simulink model "CPG_online"  (R2021b)
settings: Solver=FixedStepDiscrete  StartTime=0.0  StopTime=inf  FixedStep=Ts_cal  MaxStep=0.05  RelTol=0.5  AbsTol=0.5
model workspace (MATLAB code in the model file):
  | %---------------Critical values---------------%
  | angle_amp = pi/4; % Motor rotate amplitude, ref: pi/4
  | rotateCorrectionCoef = 1.158;
  | criticalFn = 2;
  | 
  | %------values for normalization---------------%
  | % values got by running manual gait
  | rotxNormGain = 1/0.1;
  | rotyNormGain = 1/0.05;
  | rotzNormGain = 1/0.1;
  | 
  | vxNormGain = 1/0.2;
  | vyNormGain = 1/0.2;
  | vzNormGain = 1/0.2;
  | 
  | FnNormGain = 1/15;
  | 
  | %--------values for check done---------------%
  | rotDone = pi/6;
  | legBendDone = pi/3; % actuator max bending angle
  | 
  | %---------------Robot parameters-------------%
  | % robot size
  | robot_width = 0.15;
  | robot_length = 0.22;
  | 
  | % floor parameters
  | floor_length = 2;
  | floor_width = 2;
  | 
  | % continuum actuator size
  | L_disk = 0.02944;% Disk side length (m)
  | R_w = L_disk/sqrt(3);
  | thickness_disk = 0.004; % Disk thickness (m)
  | thigh_length = 0.06;
  | R_core = 0.005; % Core radius (m)
  | length_core = 0.008; % Core length (m)
  | R_spool = 0.021; % 0.01944; % radius of the spool
  | spool_height = 0.022+0.015;
  | R_pulley = 1e-3;
  | spool_k = 0;
  | spool_d = 0;
  | hole_d = 4e-3;
  | 
  | % Material property
  | rho_PLA = 1.24e3;
  | rho = 1.19e3; % 1.19e3; % Density (kg/m^3)
  | % use rigid joints
  | Pz_stiff = 135000;
  | Pz_damping = 500;
  | S_stiff = 0.0239;
  | S_damping = 7.5e-5;
  | S_low_Bound = -20;
  | S_up_Bound = 20;
  | 
  | R_foot = 0.015; % foot radius (m)
  | 
  | % motor parameter
  | stall_T = 11.2/10; % 11.2 cm*kg, stall torque
  | t_60_deg = 0.2; % 0.09 s
  | V_nomrmal = 6; % corresponding normal voltage
  | Jr = 0.0001; %g*cm^2, robot inertia
  | 
  | % contact force
  | coef_static_friction = 0.315;
  | coef_dynamic_friction = 0.3;
  | crictic_velocity = 0.3; % m/s
  | contact_suf_stiff = 1000; % N/m
  | contact_suf_damp = 50; % N/(m/s)
  | contact_region_width = 2e-3; % m
  | spoolOpacity = 0;
  | tendonColor = [0.902 0.902 0.902];
  | tendonOpacity = 0.1;
  | 
  | % If use point masses
  | MMainFrame = 198; % g
  | MServoMotor = 50.55;
  | MMotorSupport = 12.1;
  | MSpool = 9.2;
  | 
  | % Robot total weight about 2 kg
  | MComposateLoad = 200;
  | 
  | MBuck = 40; % x2
  | MPCB_RPi = 141.3;
  | MLiBattery = 120; % x2
  | MPowerBank = 66.5;
  | isLoadVisible = 0.1;
  | 
  | 
  | MThigh = 26.7963;
  | MCore = 0.747699;
  | MDisk = 1.78642;
  | MFoot = 16.8232;
values from neighbouring files (symbols this model uses):
  A = [0 Ts; 0 1]    [MFBO_main.m]    (also in MFGP_main.m)
  A_cpg = 1    [MFBO_main.m]    (also in MFGP_main.m)
  alpha = opt_param(2)    [MFBO_main.m]    (also in MFGP_main.m)
  alpha_b_gain = opt_param(3)    [MFBO_main.m]    (also in MFGP_main.m)
  alpha_r_gain = pi    (= 3.14159265359)    [MFBO_main.m]    (also in MFGP_main.m)
  B = [0.5*Ts^2; Ts]    [MFBO_main.m]    (also in MFGP_main.m)
  C = [1 0]    [MFBO_main.m]    (also in MFGP_main.m)
  epsilon = 5    [MFBO_main.m]    (also in MFGP_main.m)
  f = 1/T    [MFBO_main.m]    (also in MFGP_main.m)
  init_state = rand(1, 8)*2 - 1    [MFBO_main.m]    (also in MFGP_main.m)
  k = 1000    [MFBO_main.m]    (also in MFGP_main.m)
  phi_vec = pi*[-1; 1; -1; 1]    [MFBO_main.m]    (also in MFGP_main.m)
  R = 0.15    [MFBO_main.m]    (also in MFGP_main.m)
  tau = 1    [MFBO_main.m]    (also in MFGP_main.m)
  Ts = 5e-2    (= 0.05)    [MFBO_main.m]    (also in MFGP_main.m)
  Ts_cal = 5e-4    (= 0.0005)    [MFBO_main.m]    (also in MFGP_main.m)
  z_l_diff = opt_param(5)    [MFBO_main.m]    (also in MFGP_main.m)
  z_l_gain = opt_param(4)    [MFBO_main.m]    (also in MFGP_main.m)
undefined symbols (not defined in the file or in its folder): DiscIntNeverNeededParam, Discrete, Time
libraries: svdutilitieslib x15, simulink x4, ctrlSharedLib x3, instrumentlib x2, aerolibanimutils x1
(part 1 of 2)
settings Model: Creator=Qinglei Ji  LastModifiedBy=4DLab5
settings SolverCC: AutoScaleAbsTol=off  MaxConsecutiveZCs=100  MaxConsecutiveMinStep=10  DaesscMode=Fast  ZeroCrossAlgorithm=Adaptive  AutoInsertRateTranBlk=on
settings DebuggingCC: AlgebraicLoopMsg=error  IgnoredZcDiagnostic=none
settings ExplorerConfigSet: InternalSimMechanicsExplorerSettings="<ExplorerConfiguration><canonicalview>default</canonicalview><AnimationSetting><BasePlaybackSpeed>1.0</BasePlaybackSpeed><PlaybackSpeedFactor>1.0</PlaybackSpeedFactor></AnimationSetting><TilePanel><TileInfo><Tiles Columns=\"1\" Count=\"1\" Rows=\"1\"><Column Weight=\"1\"/><Row Weight=\"1\"/><Tile Height=\"1\" Width=\"1\" X=\"0\" Y=\"0\"/></Tiles></TileInfo><SceneInfo><SceneViewer><BGColor><R>0.60000002384185791</R><G>0.60000002384185791</G><B>0.60000002384185791</B></BGColor><Camera><DoPerspective>off</DoPerspective><Position><X>-18.8331461547739707</X><Y>25.880517186070815</Y><Z>26.8100820833696147</Z></Position><Center><X>0.29785977478998571</X><Y>-0.293010908258582892</Y><Z>-0.346783787749327221</Z></Center><Up><X>0.517886432622382209</X><Y>-0.40389178028612327</Y><Z>0.754098848111419029</Z></Up><ViewLimDist>1</ViewLimDist><YLim>0.421333194645766129</YLim><XLim>0.456755011894746488</XLim></Camera></SceneViewer></SceneInfo></TilePanel><MechEditorPanel><Cameras/><GfxPanelCameraMap/><VideoCreator><PlaybackSpeedRatio>1.0</PlaybackSpeedRatio><FrameRate>60</FrameRate><VideoFormat>MPEG-4</VideoFormat><FrameSize>auto</FrameSize></VideoCreator></MechEditorPanel></ExplorerConfiguration>"

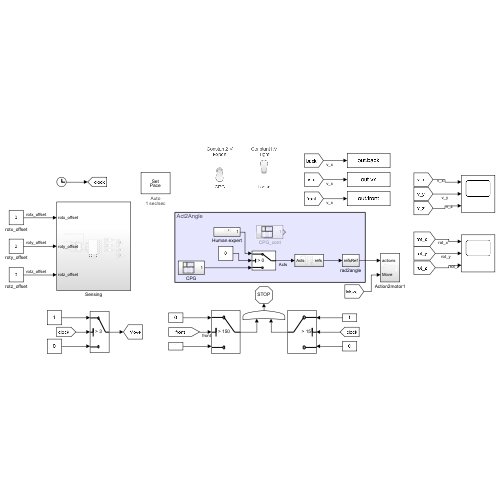
[thumbnail: Simulink's stored preview of the top-level diagram]
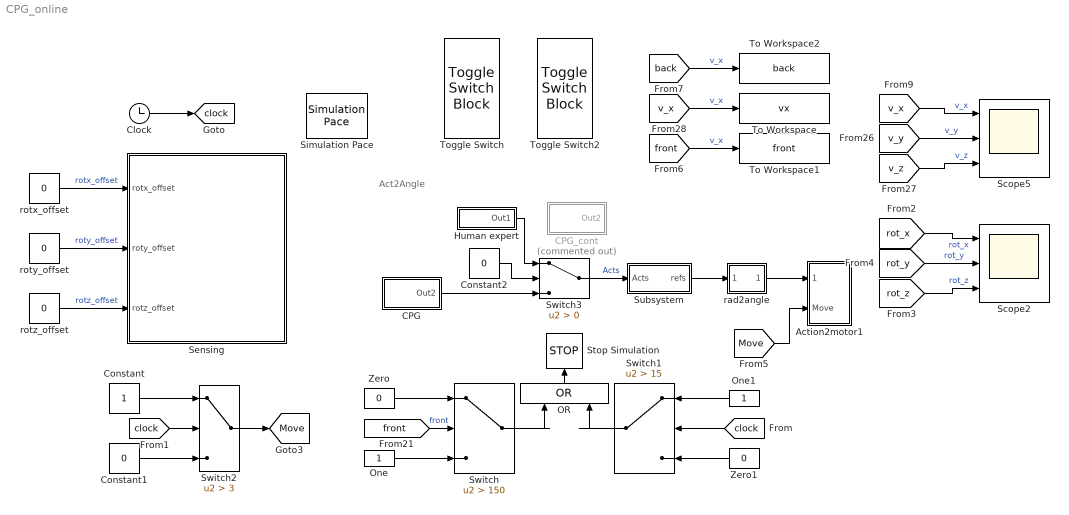
== system CPG_online ==
  note: Act2Angle
  Action2motor1 : Subsystem
  CPG : Subsystem
  CPG_cont : Subsystem  Commented=on
  Clock : Clock
  Constant : Constant
  Constant1 : Constant  Value=0
  Constant2 : Constant  Value=0
  Human expert : Subsystem
  OR : Logic  Operator=OR  IconShape=distinctive  AllPortsSameDT=off  OutDataTypeStr=boolean
  One : Constant  OutDataTypeStr=Inherit: Inherit via back propagation
  One1 : Constant  OutDataTypeStr=Inherit: Inherit via back propagation
  Scope2 : Scope  NumInputPorts=3
  Scope5 : Scope  NumInputPorts=3
  Sensing : Subsystem
  Simulation Pace : aerolibanimutils/Simulation Pace  SimulationPace=1  SleepMode=Auto  OutputPaceError=off  SampleTime=0.05
  Stop Simulation : Stop
  Subsystem : Subsystem
  Switch : Switch  Criteria=u2 > Threshold  Threshold=150
  Switch1 : Switch  Criteria=u2 > Threshold  Threshold=15
  Switch2 : Switch  Criteria=u2 > Threshold  Threshold=3
  Switch3 : Switch  Criteria=u2 > Threshold
  To Workspace : ToWorkspace  VariableName=vx  SampleTime=-1
  To Workspace1 : ToWorkspace  VariableName=front  SampleTime=-1
  To Workspace2 : ToWorkspace  VariableName=back  SampleTime=-1
  Toggle Switch : ToggleSwitchBlock
      settings: Values={{'CPG', 'Expert'}, [0 1]}
  Toggle Switch2 : ToggleSwitchBlock
      settings: Values={{'Loose', 'Tight'}, [0 1]}
  Zero : Constant  Value=0  OutDataTypeStr=Inherit: Inherit via back propagation
  Zero1 : Constant  Value=0  OutDataTypeStr=Inherit: Inherit via back propagation
  rad2angle : Subsystem
  rotx_offset : Constant  Value=0
  roty_offset : Constant  Value=0
  rotz_offset : Constant  Value=0
  tag scope: Move=global, clock=global
  wires:
  rad2angle/1(Ref) -> Action2motor1/1(actions)
  OR/1 -> Stop Simulation/1
  [front] -> Switch/2  "front"
  Zero/1 -> Switch/1
  One/1 -> Switch/3
  Switch/1 -> OR/1
  Switch1/1 -> OR/2
  Clock/1 -> [clock]
  [clock] -> Switch1/2
  Zero1/1 -> Switch1/3
  One1/1 -> Switch1/1
  [rot_y] -> Scope2/2  "rot_y"
  [rot_z] -> Scope2/3  "rot_z"
  [rot_x] -> Scope2/1  "rot_x"
  [v_z] -> Scope5/3  "v_z"
  [v_y] -> Scope5/2  "v_y"
  [v_x] -> Scope5/1  "v_x"
  [v_x] -> To Workspace/1  "v_x"
  Subsystem/1(refs) -> rad2angle/1(refs)
  Switch3/1 -> Subsystem/1(Acts)  "Acts"
  rotx_offset/1 -> Sensing/1(rotx_offset)  "rotx_offset"
  roty_offset/1 -> Sensing/2(roty_offset)  "roty_offset"
  rotz_offset/1 -> Sensing/3(rotz_offset)  "rotz_offset"
  Constant/1 -> Switch2/1
  Constant1/1 -> Switch2/3
  [clock] -> Switch2/2
  Switch2/1 -> [Move]
  [Move] -> Action2motor1/2(Move)
  Constant2/1 -> Switch3/2
  Human expert/1(Out1) -> Switch3/1
  CPG/1(Out2) -> Switch3/3
  [front] -> To Workspace1/1  "v_x"
  [back] -> To Workspace2/1  "v_x"

== system CPG_online/Action2motor1 ==
  actions : Inport
  Move : Inport  Port=2
  Add : Sum  Inputs=+-
  Constant : Constant  Value=0
  Constant1 : Constant
  Constant2 : Constant  Value=15
  Data Type Conversion2 : DataTypeConversion  OutDataTypeStr=uint8
  Display : Display
  Rate Transition : RateTransition  OutPortSampleTime=Ts
  Switch : Switch  Criteria=u2 > Threshold
  Switch1 : Switch  Criteria=u2 > Threshold
  TCP/IP Send : instrumentlib/TCP//IP Send  Priority=1  Host=192.168.0.111  Port=6666  ByteOrder=big-endian  EnableBlockingMode=on  Timeout=1  TransferDelay=on  SimulateUsing=Interpreted execution
  manual angle input2 : Subsystem
  pretighten : Subsystem
  pretighten1 : Subsystem  Commented=on
  wires:
  manual angle input2/1(Out1) -> Switch1/3
  pretighten/1(Out1) -> Add/2
  Switch1/1 -> Add/1
  Switch/1 -> pretighten/1(In1)
  Constant/1 -> Switch/3
  Constant2/1 -> Switch/1
  Data Type Conversion2/1 -> Display/1, TCP/IP Send/1
  Add/1 -> Rate Transition/1
  Constant1/1 -> Switch/2
  Move/1 -> Switch1/2
  actions/1 -> Switch1/1
  Rate Transition/1 -> Data Type Conversion2/1

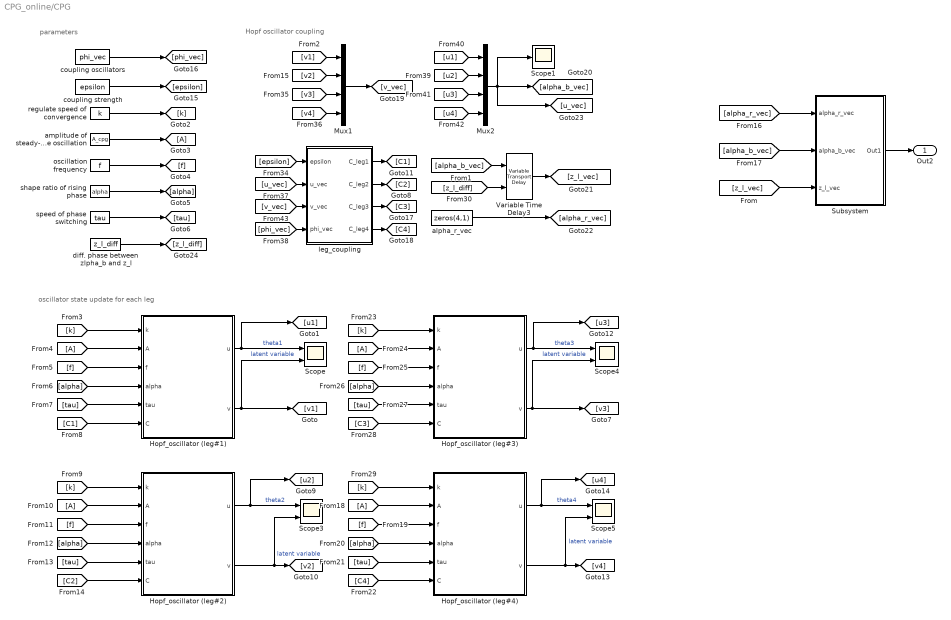
== system CPG_online/CPG ==
  note: oscillator state update for each leg
  note: Hopf oscillator coupling
  note: parameters
  Hopf_oscillator (leg#1) : Subsystem
  Hopf_oscillator (leg#2) : Subsystem
  Hopf_oscillator (leg#3) : Subsystem
  Hopf_oscillator (leg#4) : Subsystem
  Mux1 : Mux
  Mux2 : Mux
  Scope{,3..5} (4 alike) : Scope  NumInputPorts=2
  Scope1 : Scope
  Subsystem : Subsystem
  Variable Time Delay3 : VariableTransportDelay  MaximumDelay=10  MaximumPoints=2^20  FixedBuffer=on  ZeroDelay=on
  alpha_r_vec : Constant  Value=zeros(4,1)
  amplitude of steady-state oscillation : Constant  Value=A_cpg
  coupling oscillators : Constant  Value=phi_vec
  coupling strength : Constant  Value=epsilon
  diff. phase between zlpha_b and z_l : Constant  Value=z_l_diff
  leg_coupling : MATLAB Function  TreatAsAtomicUnit=on
  oscillation frequency : Constant  Value=f
  regulate speed of convergence : Constant  Value=k
  shape ratio of rising phase : Constant  Value=alpha
  speed of phase switching : Constant  Value=tau
  Out2 : Outport
  wires:
  [k] -> Hopf_oscillator (leg#4)/1(k)
  [tau] -> Hopf_oscillator (leg#3)/5(tau)
  [u4] -> Mux2/4
  [v2] -> Mux1/2
  shape ratio of rising phase/1 -> [alpha]
  [epsilon] -> leg_coupling/1(epsilon)
  [u3] -> Mux2/3
  [v_vec] -> leg_coupling/3(v_vec)
  [C2] -> Hopf_oscillator (leg#2)/6(C)
  leg_coupling/4(C_leg4) -> [C4]
  [f] -> Hopf_oscillator (leg#3)/3(f)
  Hopf_oscillator (leg#4)/1(u) -> [u4], Scope5/1  "theta4"
  Hopf_oscillator (leg#4)/2(v) -> [v4], Scope5/2  "latent variable"
  [k] -> Hopf_oscillator (leg#3)/1(k)
  leg_coupling/2(C_leg2) -> [C2]
  oscillation frequency/1 -> [f]
  [u1] -> Mux2/1
  Hopf_oscillator (leg#3)/1(u) -> [u3], Scope4/1  "theta3"
  [A] -> Hopf_oscillator (leg#3)/2(A)
  leg_coupling/3(C_leg3) -> [C3]
  [u2] -> Mux2/2
  Hopf_oscillator (leg#1)/2(v) -> [v1], Scope/2  "latent variable"
  [alpha] -> Hopf_oscillator (leg#2)/4(alpha)
  Hopf_oscillator (leg#3)/2(v) -> [v3], Scope4/2  "latent variable"
  speed of phase switching/1 -> [tau]
  [f] -> Hopf_oscillator (leg#2)/3(f)
  [tau] -> Hopf_oscillator (leg#4)/5(tau)
  [u_vec] -> leg_coupling/2(u_vec)
  [alpha] -> Hopf_oscillator (leg#3)/4(alpha)
  amplitude of steady-state oscillation/1 -> [A]
  [A] -> Hopf_oscillator (leg#1)/2(A)
  [A] -> Hopf_oscillator (leg#2)/2(A)
  leg_coupling/1(C_leg1) -> [C1]
  Mux2/1 -> [u_vec], [alpha_b_vec], Scope1/1
  Hopf_oscillator (leg#2)/1(u) -> [u2], Scope3/1  "theta2"
  [v4] -> Mux1/4
  [f] -> Hopf_oscillator (leg#4)/3(f)
  [C4] -> Hopf_oscillator (leg#4)/6(C)
  [C3] -> Hopf_oscillator (leg#3)/6(C)
  [tau] -> Hopf_oscillator (leg#1)/5(tau)
  coupling strength/1 -> [epsilon]
  [A] -> Hopf_oscillator (leg#4)/2(A)
  [k] -> Hopf_oscillator (leg#2)/1(k)
  [alpha] -> Hopf_oscillator (leg#4)/4(alpha)
  [v3] -> Mux1/3
  [k] -> Hopf_oscillator (leg#1)/1(k)
  [phi_vec] -> leg_coupling/4(phi_vec)
  [C1] -> Hopf_oscillator (leg#1)/6(C)
  [v1] -> Mux1/1
  Mux1/1 -> [v_vec]
  [tau] -> Hopf_oscillator (leg#2)/5(tau)
  [f] -> Hopf_oscillator (leg#1)/3(f)
  regulate speed of convergence/1 -> [k]
  Hopf_oscillator (leg#2)/2(v) -> [v2], Scope3/2  "latent variable"
  Hopf_oscillator (leg#1)/1(u) -> [u1], Scope/1  "theta1"
  [alpha] -> Hopf_oscillator (leg#1)/4(alpha)
  coupling oscillators/1 -> [phi_vec]
  [alpha_b_vec] -> Variable Time Delay3/1
  [z_l_diff] -> Variable Time Delay3/2
  Variable Time Delay3/1 -> [z_l_vec]
  alpha_r_vec/1 -> [alpha_r_vec]
  [alpha_r_vec] -> Subsystem/1(alpha_r_vec)
  [alpha_b_vec] -> Subsystem/2(alpha_b_vec)
  [z_l_vec] -> Subsystem/3(z_l_vec)
  Subsystem/1(Out1) -> Out2/1
  diff. phase between zlpha_b and z_l/1 -> [z_l_diff]

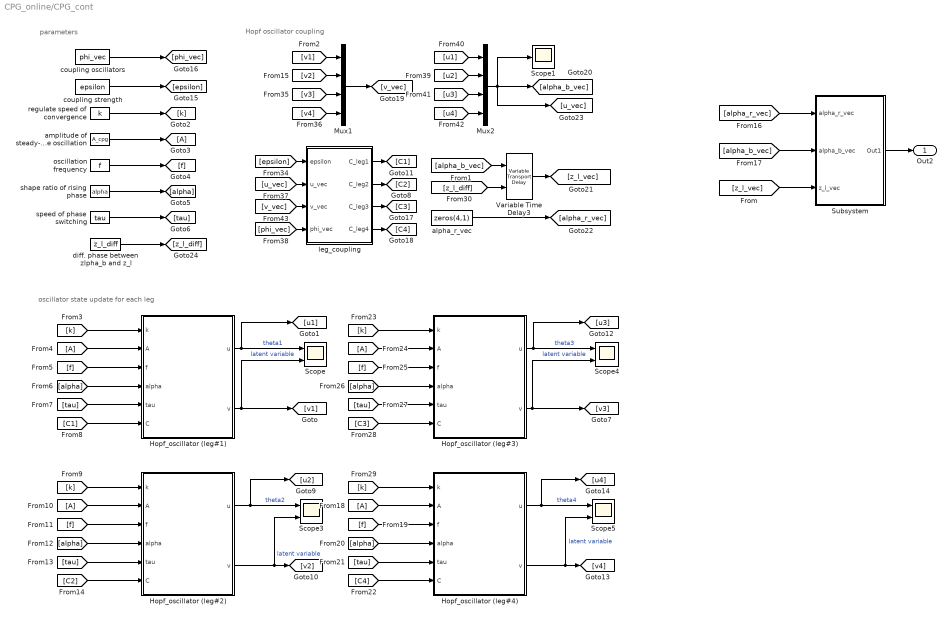
== system CPG_online/CPG_cont ==
  note: oscillator state update for each leg
  note: Hopf oscillator coupling
  note: parameters
  Hopf_oscillator (leg#1) : Subsystem
  Hopf_oscillator (leg#2) : Subsystem
  Hopf_oscillator (leg#3) : Subsystem
  Hopf_oscillator (leg#4) : Subsystem
  Mux1 : Mux
  Mux2 : Mux
  Scope{,3..5} (4 alike) : Scope  NumInputPorts=2
  Scope1 : Scope
  Subsystem : Subsystem
  Variable Time Delay3 : VariableTransportDelay  MaximumDelay=10  MaximumPoints=4096  ZeroDelay=on
  alpha_r_vec : Constant  Value=zeros(4,1)
  amplitude of steady-state oscillation : Constant  Value=A_cpg
  coupling oscillators : Constant  Value=phi_vec
  coupling strength : Constant  Value=epsilon
  diff. phase between zlpha_b and z_l : Constant  Value=z_l_diff
  leg_coupling : MATLAB Function  TreatAsAtomicUnit=on
  oscillation frequency : Constant  Value=f
  regulate speed of convergence : Constant  Value=k
  shape ratio of rising phase : Constant  Value=alpha
  speed of phase switching : Constant  Value=tau
  Out2 : Outport
  wires:
  [k] -> Hopf_oscillator (leg#4)/1(k)
  [tau] -> Hopf_oscillator (leg#3)/5(tau)
  [u4] -> Mux2/4
  [v2] -> Mux1/2
  shape ratio of rising phase/1 -> [alpha]
  [epsilon] -> leg_coupling/1(epsilon)
  [u3] -> Mux2/3
  [v_vec] -> leg_coupling/3(v_vec)
  [C2] -> Hopf_oscillator (leg#2)/6(C)
  leg_coupling/4(C_leg4) -> [C4]
  [f] -> Hopf_oscillator (leg#3)/3(f)
  Hopf_oscillator (leg#4)/1(u) -> [u4], Scope5/1  "theta4"
  Hopf_oscillator (leg#4)/2(v) -> [v4], Scope5/2  "latent variable"
  [k] -> Hopf_oscillator (leg#3)/1(k)
  leg_coupling/2(C_leg2) -> [C2]
  oscillation frequency/1 -> [f]
  [u1] -> Mux2/1
  Hopf_oscillator (leg#3)/1(u) -> [u3], Scope4/1  "theta3"
  [A] -> Hopf_oscillator (leg#3)/2(A)
  leg_coupling/3(C_leg3) -> [C3]
  [u2] -> Mux2/2
  Hopf_oscillator (leg#1)/2(v) -> [v1], Scope/2  "latent variable"
  [alpha] -> Hopf_oscillator (leg#2)/4(alpha)
  Hopf_oscillator (leg#3)/2(v) -> [v3], Scope4/2  "latent variable"
  speed of phase switching/1 -> [tau]
  [f] -> Hopf_oscillator (leg#2)/3(f)
  [tau] -> Hopf_oscillator (leg#4)/5(tau)
  [u_vec] -> leg_coupling/2(u_vec)
  [alpha] -> Hopf_oscillator (leg#3)/4(alpha)
  amplitude of steady-state oscillation/1 -> [A]
  [A] -> Hopf_oscillator (leg#1)/2(A)
  [A] -> Hopf_oscillator (leg#2)/2(A)
  leg_coupling/1(C_leg1) -> [C1]
  Mux2/1 -> [u_vec], [alpha_b_vec], Scope1/1
  Hopf_oscillator (leg#2)/1(u) -> [u2], Scope3/1  "theta2"
  [v4] -> Mux1/4
  [f] -> Hopf_oscillator (leg#4)/3(f)
  [C4] -> Hopf_oscillator (leg#4)/6(C)
  [C3] -> Hopf_oscillator (leg#3)/6(C)
  [tau] -> Hopf_oscillator (leg#1)/5(tau)
  coupling strength/1 -> [epsilon]
  [A] -> Hopf_oscillator (leg#4)/2(A)
  [k] -> Hopf_oscillator (leg#2)/1(k)
  [alpha] -> Hopf_oscillator (leg#4)/4(alpha)
  [v3] -> Mux1/3
  [k] -> Hopf_oscillator (leg#1)/1(k)
  [phi_vec] -> leg_coupling/4(phi_vec)
  [C1] -> Hopf_oscillator (leg#1)/6(C)
  [v1] -> Mux1/1
  Mux1/1 -> [v_vec]
  [tau] -> Hopf_oscillator (leg#2)/5(tau)
  [f] -> Hopf_oscillator (leg#1)/3(f)
  regulate speed of convergence/1 -> [k]
  Hopf_oscillator (leg#2)/2(v) -> [v2], Scope3/2  "latent variable"
  Hopf_oscillator (leg#1)/1(u) -> [u1], Scope/1  "theta1"
  [alpha] -> Hopf_oscillator (leg#1)/4(alpha)
  coupling oscillators/1 -> [phi_vec]
  [alpha_b_vec] -> Variable Time Delay3/1
  [z_l_diff] -> Variable Time Delay3/2
  Variable Time Delay3/1 -> [z_l_vec]
  alpha_r_vec/1 -> [alpha_r_vec]
  [alpha_r_vec] -> Subsystem/1(alpha_r_vec)
  [alpha_b_vec] -> Subsystem/2(alpha_b_vec)
  [z_l_vec] -> Subsystem/3(z_l_vec)
  Subsystem/1(Out1) -> Out2/1
  diff. phase between zlpha_b and z_l/1 -> [z_l_diff]

== system CPG_online/Human expert ==
  Constant : Constant  Value=0+0.4  SampleTime=Ts
  Constant1 : Constant  Value=0  SampleTime=Ts
  Constant2 : Constant  Value=0+0.4  SampleTime=Ts
  Mux1 : Mux  Inputs=3
  Mux2 : Mux
  Mux3 : Mux  Commented=on  Inputs=3
  Sine Wave : Sin  Frequency=2*pi/0.8  SampleTime=Ts
  Sine Wave1 : Sin  Frequency=2*pi/0.8  Phase=pi  SampleTime=Ts
  Variable Time Delay : VariableTransportDelay  MaximumDelay=10  MaximumPoints=2^15  ZeroDelay=on
  Variable Time Delay1 : VariableTransportDelay  MaximumDelay=10  MaximumPoints=2^15  ZeroDelay=on
  Variable Time Delay2 : VariableTransportDelay  MaximumDelay=10  MaximumPoints=2^15  ZeroDelay=on
  alpha_b : simulink/Sources/Repeating Sequence  Commented=on  rep_seq_t=[0 0.2 0.4 0.6 0.8]  rep_seq_y=[0 1 0 -1 0]
  alpha_b1 : simulink/Sources/Repeating Sequence  Commented=on  rep_seq_t=[0 0.2 0.4 0.6 0.8]  rep_seq_y=[0 -1 0 1 0]
  alpha_r : Constant  Value=0
  alpha_r1 : Constant  Commented=on  Value=0
  z_l : simulink/Sources/Repeating Sequence  Commented=on  rep_seq_t=[0 0.2 0.4 0.6 0.8]  rep_seq_y=[-1 1 1 1 -1]
  z_l1 : simulink/Sources/Repeating Sequence  Commented=on  rep_seq_t=[0 0.2 0.4 0.6 0.8]  rep_seq_y=[1 1 -1 1 1]
  Out1 : Outport
  wires:
  Mux2/1 -> Out1/1
  Mux1/1 -> Variable Time Delay2/1, Variable Time Delay/1, Mux2/1, Variable Time Delay1/1
  Sine Wave/1 -> Mux1/2  "alpha_b_Ref"
  alpha_r/1 -> Mux1/1  "alpha_r_Ref"
  Sine Wave1/1 -> Mux1/3  "z_l_Ref"
  Constant/1 -> Variable Time Delay/2
  z_l1/1 -> Mux3/3  "z_l_Ref"
  alpha_r1/1 -> Mux3/1  "alpha_r_Ref"
  alpha_b1/1 -> Mux3/2  "alpha_b_Ref"
  Variable Time Delay/1 -> Mux2/2
  Constant1/1 -> Variable Time Delay1/2
  Variable Time Delay2/1 -> Mux2/4
  Variable Time Delay1/1 -> Mux2/3
  Constant2/1 -> Variable Time Delay2/2

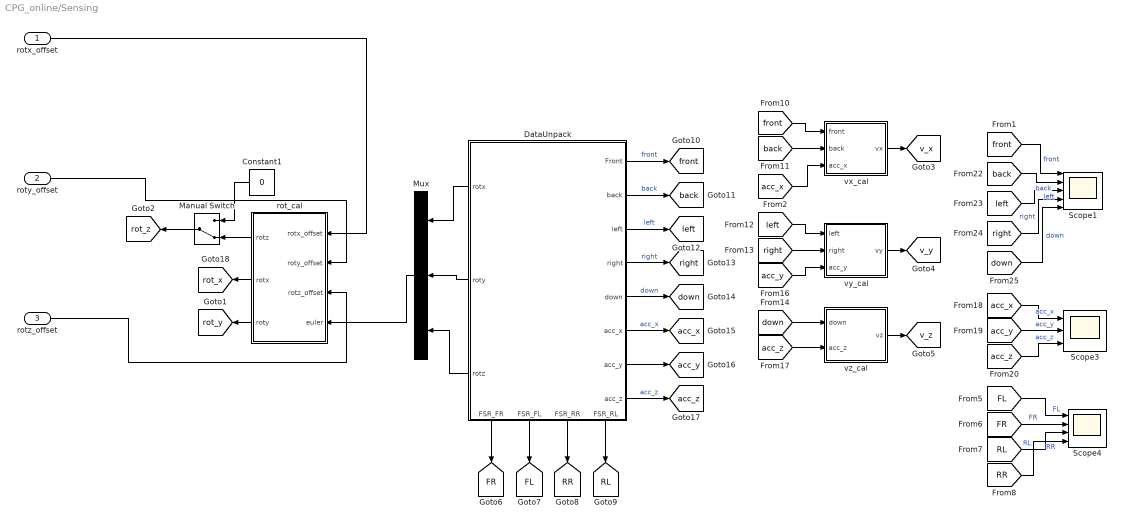
== system CPG_online/Sensing ==
  rotx_offset : Inport
  roty_offset : Inport  Port=2
  rotz_offset : Inport  Port=3
  Constant1 : Constant  Value=0
  DataUnpack : Subsystem
      settings: PortSchema="{\"entries\":[{\"content\":{\"sides\":[{\"content\":{\"connectorIds\":[\"Out13\",\"Out14\",\"Out15\"]},\"type\":\"ConnectorPlacement.EquallySpacedRectSide\",\"uuid\":\"921b036b-a103-4c29-98a4-1e13be366f27\"},{\"content\":{\"connectorIds\":[\"Out1\",\"Out2\",\"Out3\",\"Out4\",\"Out5\",\"Out6\",\"Out7\",\"Out8\"],\"side\":\"RIGHT\"},\"type\":\"ConnectorPlacement.EquallySpacedRectSide\",\"uuid\":\"743cc973-2ca6-4eb4-ab94-a827ba3cd866\"},{\"content\":{\"side\":\"TOP\"},\"type\":\"ConnectorPlacement.EquallySpacedRectSide\",\"uuid\":\"9eb642df-d260-4317-8a72-bd8569bebf98\"},{\"content\":{\"connectorIds\":[\"Out9\",\"Out10\",\"Out11\",\"Out12\"],\"side\":\"BOTTOM\"},\"type\":\"ConnectorPlacement.EquallySpacedRectSide\",\"uuid\":\"da7ab237-c829-42b0-bbc7-f99a364eb64c\"}]},\"type\":\"ConnectorPlacement.EquallySpacedConnector\",\"uuid\":\"aa8a793e-4baf-4a67-be1f-284a705b408b\"}],\"packageUris\":[\"http://schema.mathworks.com/mf0/Connector/R2020b\"],\"version\":\"1.0\"}"
  Manual Switch : ManualSwitch  CurrentSetting=0
  Mux : Mux  Inputs=3
  Scope1 : Scope  NumInputPorts=5
  Scope3 : Scope  NumInputPorts=3
  Scope4 : Scope  NumInputPorts=4
  rot_cal : Subsystem
  vx_cal : Subsystem
  vy_cal : Subsystem
  vz_cal : Subsystem
  tag scope: FL=global, FR=global, RL=global, RR=global, acc_x=global, acc_y=global, acc_z=global, back=global, down=global, front=global, left=global, right=global, rot_x=global, rot_y=global, rot_z=global, v_x=global, v_y=global, v_z=global
  wires:
  DataUnpack/10(FSR_FL) -> [FL]
  DataUnpack/4(right) -> [right]  "right"
  [RR] -> Scope4/4  "RR"
  [acc_y] -> Scope3/2  "acc_y"
  [FR] -> Scope4/2  "FR"
  [back] -> Scope1/2  "back"
  [RL] -> Scope4/3  "RL"
  [front] -> Scope1/1  "front"
  [front] -> vx_cal/1(front)
  DataUnpack/2(back) -> [back]  "back"
  DataUnpack/11(FSR_RR) -> [RR]
  [FL] -> Scope4/1  "FL"
  [right] -> Scope1/4  "right"
  rot_cal/3(roty) -> [rot_y]
  rot_cal/1(rotz) -> Manual Switch/2
  DataUnpack/12(FSR_RL) -> [RL]
  DataUnpack/8(acc_z) -> [acc_z]  "acc_z"
  rotx_offset/1 -> rot_cal/1(rotx_offset)
  vy_cal/1(vy) -> [v_y]
  DataUnpack/9(FSR_FR) -> [FR]
  DataUnpack/7(acc_y) -> [acc_y]
  Mux/1 -> rot_cal/4(euler)
  DataUnpack/15(rotz) -> Mux/3
  DataUnpack/6(acc_x) -> [acc_x]  "acc_x"
  DataUnpack/13(rotx) -> Mux/1
  DataUnpack/14(roty) -> Mux/2
  vz_cal/1(vz) -> [v_z]
  [back] -> vx_cal/2(back)
  DataUnpack/5(down) -> [down]  "down"
  DataUnpack/3(left) -> [left]  "left"
  DataUnpack/1(Front) -> [front]  "front"
  rotz_offset/1 -> rot_cal/3(rotz_offset)
  [acc_x] -> Scope3/1  "acc_x"
  [acc_z] -> Scope3/3  "acc_z"
  Manual Switch/1 -> [rot_z]
  Constant1/1 -> Manual Switch/1
  rot_cal/2(rotx) -> [rot_x]
  vx_cal/1(vx) -> [v_x]
  [left] -> Scope1/3  "left"
  [down] -> Scope1/5  "down"
  [acc_z] -> vz_cal/2(acc_z)
  [acc_y] -> vy_cal/3(acc_y)
  [right] -> vy_cal/2(right)
  roty_offset/1 -> rot_cal/2(roty_offset)
  [down] -> vz_cal/1(down)
  [left] -> vy_cal/1(left)
  [acc_x] -> vx_cal/3(acc_x)

== system CPG_online/Subsystem ==
  Acts : Inport
  Demux : Demux
  FL : Subsystem
  FR : Subsystem
  Mux : Mux
  RL : Subsystem
  RR : Subsystem
  To Workspace : ToWorkspace  VariableName=action  SaveFormat=Structure  SampleTime=Ts
      settings: Save2DSignal=2-D array (concatenate along first dimension)
  refs : Outport
  wires:
  Demux/4 -> RR/1(act)
  FR/1(angle) -> Mux/1
  Demux/2 -> FL/1(act)
  Demux/3 -> RL/1(act)
  Demux/1 -> FR/1(act)
  FL/1(angle) -> Mux/2
  Acts/1 -> Demux/1, To Workspace/1
  Mux/1 -> refs/1
  RR/1(angle) -> Mux/3
  RL/1(angle) -> Mux/4

== system CPG_online/rad2angle ==
  refs : Inport
  Constant10 : Constant  Value=90
  Gain : Gain  Gain=180/pi
  Sum : Sum
  Ref : Outport
  wires:
  Constant10/1 -> Sum/2
  Sum/1 -> Ref/1
  refs/1 -> Gain/1
  Gain/1 -> Sum/1

== system CPG_online/Action2motor1/manual angle input2 ==
  Constant{,3..13} (12 alike) : Constant  Value=90  SampleTime=-1
  Mux : Mux  Inputs=12
  Out1 : Outport
  wires:
  Constant3/1 -> Mux/2
  Constant11/1 -> Mux/10
  Constant9/1 -> Mux/8
  Constant8/1 -> Mux/7
  Constant/1 -> Mux/1
  Constant4/1 -> Mux/3
  Constant10/1 -> Mux/9
  Constant5/1 -> Mux/4
  Constant7/1 -> Mux/6
  Constant13/1 -> Mux/12
  Constant12/1 -> Mux/11
  Constant6/1 -> Mux/5
  Mux/1 -> Out1/1

== system CPG_online/Action2motor1/pretighten ==
  In1 : Inport
  Add : Sum  Inputs=+++
  Constant : Constant  Value=0
  Constant10 : Constant  Value=9  SampleTime=-1
  Constant11 : Constant  Value=4  SampleTime=-1
  Constant12 : Constant  Value=0  SampleTime=-1
  Constant13 : Constant  Value=10  SampleTime=-1
  Constant16 : Constant  SampleTime=-1
  Constant17 : Constant  Value=8  SampleTime=-1
  Constant4 : Constant  Value=10  SampleTime=-1
  Constant5 : Constant  Value=-7  SampleTime=-1
  Constant6 : Constant  Value=-3  SampleTime=-1
  Constant7 : Constant  Value=5  SampleTime=-1
  Constant8 : Constant  Value=-2  SampleTime=-1
  Constant9 : Constant  Value=12  SampleTime=-1
  Mux : Mux  Inputs=12
  Out1 : Outport
  wires:
  Constant12/1 -> Mux/11
  Constant6/1 -> Mux/5
  Constant9/1 -> Mux/8
  Constant4/1 -> Mux/3
  Constant13/1 -> Mux/12
  Constant7/1 -> Mux/6
  Constant5/1 -> Mux/4
  Mux/1 -> Add/2
  Constant10/1 -> Mux/9
  Constant8/1 -> Mux/7
  Constant11/1 -> Mux/10
  Constant17/1 -> Mux/2
  Constant/1 -> Add/1
  Constant16/1 -> Mux/1
  Add/1 -> Out1/1
  In1/1 -> Add/3

== system CPG_online/Action2motor1/pretighten1 ==
  In1 : Inport
  Add : Sum  Inputs=+++
  Constant : Constant  Value=0
  Constant10 : Constant  Value=5  SampleTime=-1
  Constant{8,11..12,16} (4 alike) : Constant  Value=0  SampleTime=-1
  Constant13 : Constant  Value=3  SampleTime=-1
  Constant17 : Constant  Value=3  SampleTime=-1
  Constant4 : Constant  Value=10  SampleTime=-1
  Constant5 : Constant  Value=5  SampleTime=-1
  Constant6 : Constant  Value=-2  SampleTime=-1
  Constant7 : Constant  Value=4  SampleTime=-1
  Constant9 : Constant  Value=5  SampleTime=-1
  Mux : Mux  Inputs=12
  Out1 : Outport
  wires:
  Constant12/1 -> Mux/11
  Constant6/1 -> Mux/5
  Constant9/1 -> Mux/8
  Constant4/1 -> Mux/3
  Constant13/1 -> Mux/12
  Constant7/1 -> Mux/6
  Constant5/1 -> Mux/4
  Mux/1 -> Add/2
  Constant10/1 -> Mux/9
  Constant8/1 -> Mux/7
  Constant11/1 -> Mux/10
  Constant17/1 -> Mux/2
  Constant/1 -> Add/1
  Constant16/1 -> Mux/1
  Add/1 -> Out1/1
  In1/1 -> Add/3

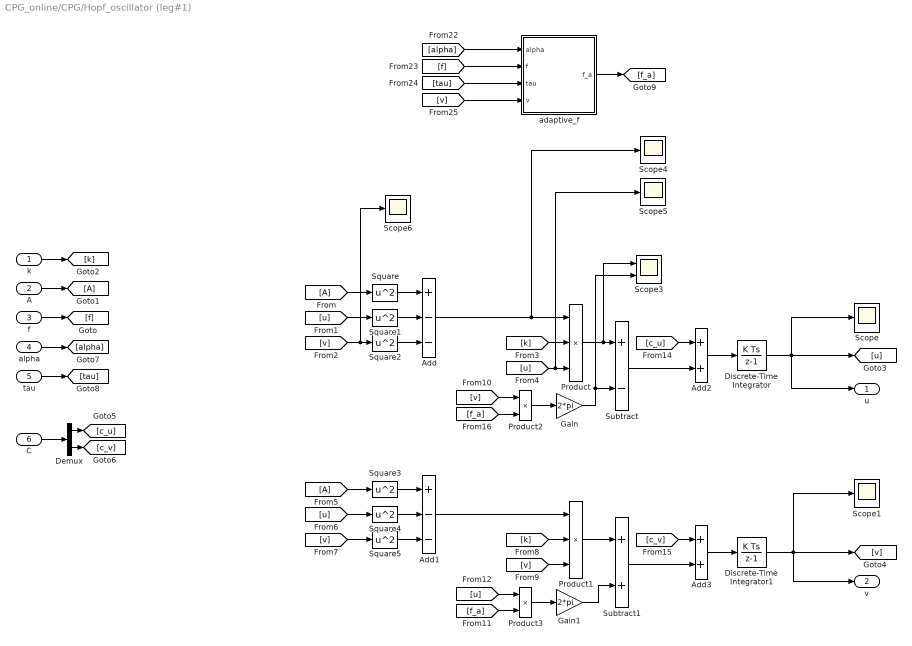
== system CPG_online/CPG/Hopf_oscillator (leg#1) ==
  k : Inport
  A : Inport  Port=2
  f : Inport  Port=3
  alpha : Inport  Port=4
  tau : Inport  Port=5
  C : Inport  Port=6
  Add : Sum  Inputs=+--
  Add1 : Sum  Inputs=+--
  Add2 : Sum
  Add3 : Sum
  Demux : Demux  Outputs=2
  Discrete-Time Integrator : DiscreteIntegrator  InitialCondition=init_state(1)  SampleTime=Ts_cal  ICPrevOutput=DiscIntNeverNeededParam  ICPrevScaledInput=DiscIntNeverNeededParam
  Discrete-Time Integrator1 : DiscreteIntegrator  InitialCondition=init_state(2)  SampleTime=Ts_cal  ICPrevOutput=DiscIntNeverNeededParam  ICPrevScaledInput=DiscIntNeverNeededParam
  Gain : Gain  Gain=2*pi
  Gain1 : Gain  Gain=2*pi
  Product : Product  Inputs=3
  Product1 : Product  Inputs=3
  Product2 : Product
  Product3 : Product
  Scope{,1,4..6} (5 alike) : Scope
  Scope3 : Scope  NumInputPorts=2
  Square{,1..5} (6 alike) : Math  Operator=square  SaturateOnIntegerOverflow=on
  Subtract : Sum  Inputs=+-
  Subtract1 : Sum
  adaptive_f : MATLAB Function  TreatAsAtomicUnit=on
  u : Outport
  v : Outport  Port=2
  wires:
  Discrete-Time Integrator/1 -> Scope/1, [u], u/1
  f/1 -> [f]
  A/1 -> [A]
  k/1 -> [k]
  [A] -> Square/1
  [u] -> Square1/1
  [v] -> Scope6/1, Square2/1
  Square2/1 -> Add/3
  Square1/1 -> Add/2
  Square/1 -> Add/1
  [k] -> Product/2
  [u] -> Scope5/1, Product/3
  Product/1 -> Scope3/1, Subtract/1
  Square3/1 -> Add1/1
  Square4/1 -> Add1/2
  Square5/1 -> Add1/3
  [v] -> Product1/3
  Product1/1 -> Subtract1/1
  [v] -> Square5/1
  [A] -> Square3/1
  [u] -> Square4/1
  [k] -> Product1/2
  [v] -> Product2/1
  [f_a] -> Product2/2
  Product2/1 -> Gain/1
  Gain/1 -> Scope3/2, Subtract/2
  [u] -> Product3/1
  Product3/1 -> Gain1/1
  [f_a] -> Product3/2
  Gain1/1 -> Subtract1/2
  Subtract/1 -> Add2/2
  C/1 -> Demux/1
  Demux/1 -> [c_u]
  Demux/2 -> [c_v]
  [c_u] -> Add2/1
  Subtract1/1 -> Add3/2
  [c_v] -> Add3/1
  Add3/1 -> Discrete-Time Integrator1/1
  alpha/1 -> [alpha]
  tau/1 -> [tau]
  [alpha] -> adaptive_f/1(alpha)
  [f] -> adaptive_f/2(f)
  [tau] -> adaptive_f/3(tau)
  [v] -> adaptive_f/4(v)
  adaptive_f/1(f_a) -> [f_a]
  Discrete-Time Integrator1/1 -> Scope1/1, [v], v/1
  Add2/1 -> Discrete-Time Integrator/1
  Add/1 -> Scope4/1, Product/1
  Add1/1 -> Product1/1

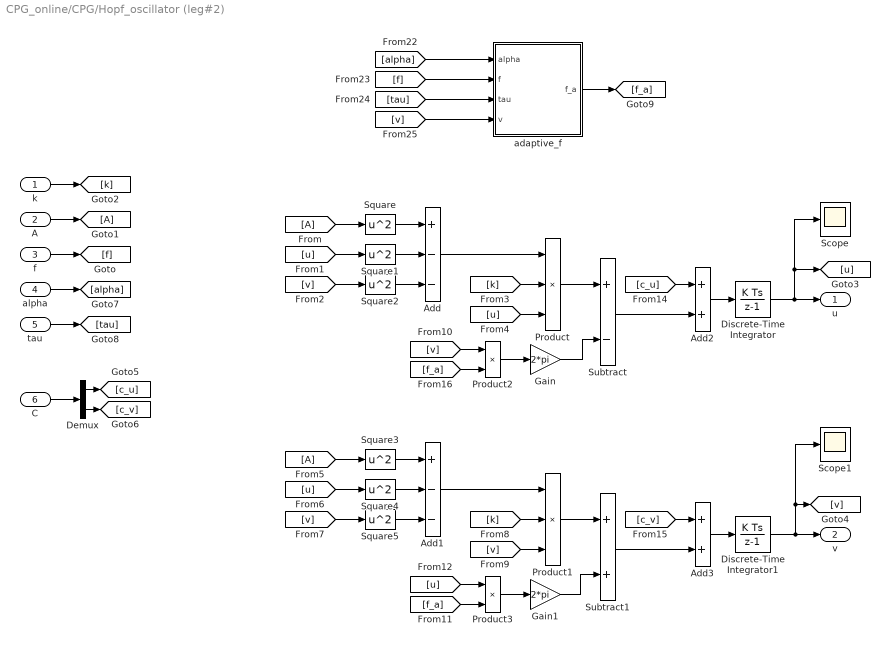
== system CPG_online/CPG/Hopf_oscillator (leg#2) ==
  k : Inport
  A : Inport  Port=2
  f : Inport  Port=3
  alpha : Inport  Port=4
  tau : Inport  Port=5
  C : Inport  Port=6
  Add : Sum  Inputs=+--
  Add1 : Sum  Inputs=+--
  Add2 : Sum
  Add3 : Sum
  Demux : Demux  Outputs=2
  Discrete-Time Integrator : DiscreteIntegrator  InitialCondition=init_state(3)  SampleTime=Ts_cal  ICPrevOutput=DiscIntNeverNeededParam  ICPrevScaledInput=DiscIntNeverNeededParam
  Discrete-Time Integrator1 : DiscreteIntegrator  InitialCondition=init_state(4)  SampleTime=Ts_cal  ICPrevOutput=DiscIntNeverNeededParam  ICPrevScaledInput=DiscIntNeverNeededParam
  Gain : Gain  Gain=2*pi
  Gain1 : Gain  Gain=2*pi
  Product : Product  Inputs=3
  Product1 : Product  Inputs=3
  Product2 : Product
  Product3 : Product
  Scope : Scope
  Scope1 : Scope
  Square{,1..5} (6 alike) : Math  Operator=square  SaturateOnIntegerOverflow=on
  Subtract : Sum  Inputs=+-
  Subtract1 : Sum
  adaptive_f : MATLAB Function  TreatAsAtomicUnit=on
  u : Outport
  v : Outport  Port=2
  wires:
  f/1 -> [f]
  A/1 -> [A]
  k/1 -> [k]
  [A] -> Square/1
  [u] -> Square1/1
  [v] -> Square2/1
  Square2/1 -> Add/3
  Square1/1 -> Add/2
  Square/1 -> Add/1
  Add/1 -> Product/1
  [k] -> Product/2
  [u] -> Product/3
  Product/1 -> Subtract/1
  Square3/1 -> Add1/1
  Square4/1 -> Add1/2
  Square5/1 -> Add1/3
  [v] -> Product1/3
  Product1/1 -> Subtract1/1
  [v] -> Square5/1
  [A] -> Square3/1
  [u] -> Square4/1
  Add1/1 -> Product1/1
  [k] -> Product1/2
  [v] -> Product2/1
  [f_a] -> Product2/2
  Product2/1 -> Gain/1
  Gain/1 -> Subtract/2
  [u] -> Product3/1
  Product3/1 -> Gain1/1
  [f_a] -> Product3/2
  Gain1/1 -> Subtract1/2
  Subtract/1 -> Add2/2
  C/1 -> Demux/1
  Demux/1 -> [c_u]
  Demux/2 -> [c_v]
  [c_u] -> Add2/1
  Add2/1 -> Discrete-Time Integrator/1
  Subtract1/1 -> Add3/2
  [c_v] -> Add3/1
  alpha/1 -> [alpha]
  tau/1 -> [tau]
  [alpha] -> adaptive_f/1(alpha)
  [f] -> adaptive_f/2(f)
  [tau] -> adaptive_f/3(tau)
  [v] -> adaptive_f/4(v)
  adaptive_f/1(f_a) -> [f_a]
  Discrete-Time Integrator/1 -> u/1, Scope/1, [u]
  Discrete-Time Integrator1/1 -> v/1, Scope1/1, [v]
  Add3/1 -> Discrete-Time Integrator1/1

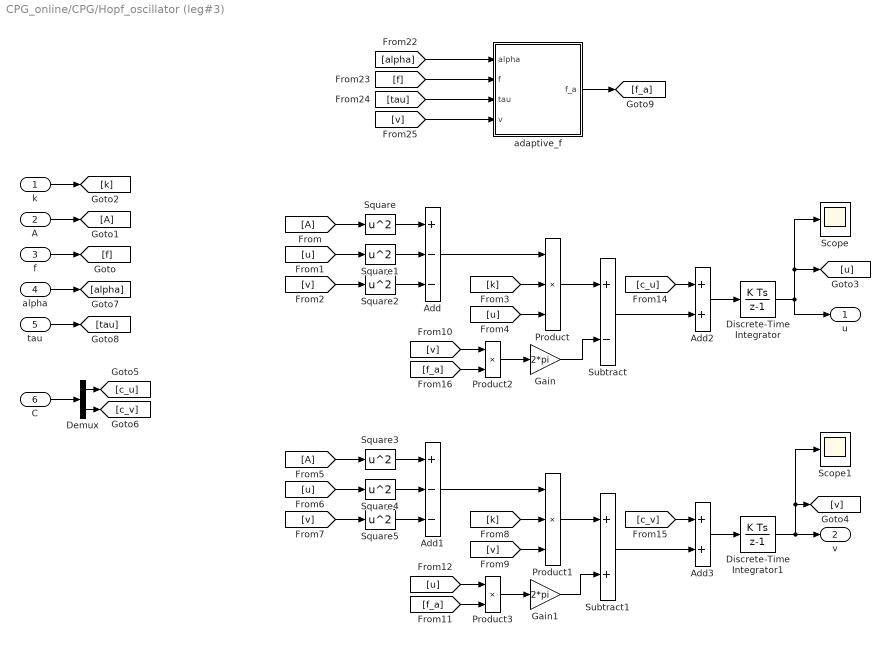
== system CPG_online/CPG/Hopf_oscillator (leg#3) ==
  k : Inport
  A : Inport  Port=2
  f : Inport  Port=3
  alpha : Inport  Port=4
  tau : Inport  Port=5
  C : Inport  Port=6
  Add : Sum  Inputs=+--
  Add1 : Sum  Inputs=+--
  Add2 : Sum
  Add3 : Sum
  Demux : Demux  Outputs=2
  Discrete-Time Integrator : DiscreteIntegrator  InitialCondition=init_state(5)  SampleTime=Ts_cal  ICPrevOutput=DiscIntNeverNeededParam  ICPrevScaledInput=DiscIntNeverNeededParam
  Discrete-Time Integrator1 : DiscreteIntegrator  InitialCondition=init_state(6)  SampleTime=Ts_cal  ICPrevOutput=DiscIntNeverNeededParam  ICPrevScaledInput=DiscIntNeverNeededParam
  Gain : Gain  Gain=2*pi
  Gain1 : Gain  Gain=2*pi
  Product : Product  Inputs=3
  Product1 : Product  Inputs=3
  Product2 : Product
  Product3 : Product
  Scope : Scope
  Scope1 : Scope
  Square{,1..5} (6 alike) : Math  Operator=square  SaturateOnIntegerOverflow=on
  Subtract : Sum  Inputs=+-
  Subtract1 : Sum
  adaptive_f : MATLAB Function  TreatAsAtomicUnit=on
  u : Outport
  v : Outport  Port=2
  wires:
  Discrete-Time Integrator/1 -> Scope/1, [u], u/1
  f/1 -> [f]
  A/1 -> [A]
  k/1 -> [k]
  [A] -> Square/1
  [u] -> Square1/1
  [v] -> Square2/1
  Square2/1 -> Add/3
  Square1/1 -> Add/2
  Square/1 -> Add/1
  Add/1 -> Product/1
  [k] -> Product/2
  [u] -> Product/3
  Product/1 -> Subtract/1
  Square3/1 -> Add1/1
  Square4/1 -> Add1/2
  Square5/1 -> Add1/3
  [v] -> Product1/3
  Product1/1 -> Subtract1/1
  [v] -> Square5/1
  [A] -> Square3/1
  [u] -> Square4/1
  Add1/1 -> Product1/1
  [k] -> Product1/2
  [v] -> Product2/1
  [f_a] -> Product2/2
  Product2/1 -> Gain/1
  Gain/1 -> Subtract/2
  [u] -> Product3/1
  Product3/1 -> Gain1/1
  [f_a] -> Product3/2
  Gain1/1 -> Subtract1/2
  Subtract/1 -> Add2/2
  C/1 -> Demux/1
  Demux/1 -> [c_u]
  Demux/2 -> [c_v]
  [c_u] -> Add2/1
  Add2/1 -> Discrete-Time Integrator/1
  Subtract1/1 -> Add3/2
  [c_v] -> Add3/1
  Add3/1 -> Discrete-Time Integrator1/1
  alpha/1 -> [alpha]
  tau/1 -> [tau]
  [alpha] -> adaptive_f/1(alpha)
  [f] -> adaptive_f/2(f)
  [tau] -> adaptive_f/3(tau)
  [v] -> adaptive_f/4(v)
  adaptive_f/1(f_a) -> [f_a]
  Discrete-Time Integrator1/1 -> v/1, Scope1/1, [v]

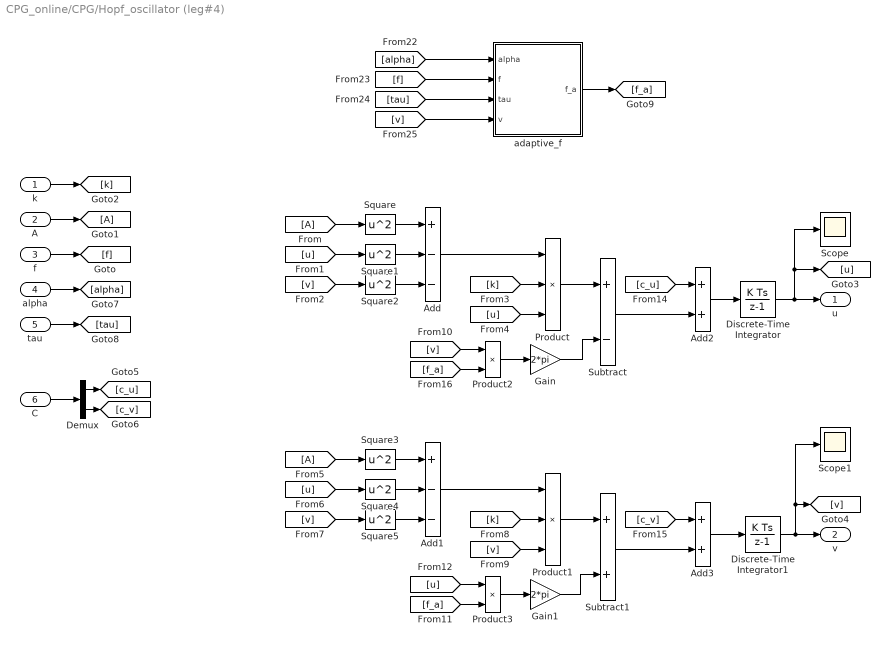
== system CPG_online/CPG/Hopf_oscillator (leg#4) ==
  k : Inport
  A : Inport  Port=2
  f : Inport  Port=3
  alpha : Inport  Port=4
  tau : Inport  Port=5
  C : Inport  Port=6
  Add : Sum  Inputs=+--
  Add1 : Sum  Inputs=+--
  Add2 : Sum
  Add3 : Sum
  Demux : Demux  Outputs=2
  Discrete-Time Integrator : DiscreteIntegrator  InitialCondition=init_state(7)  SampleTime=Ts_cal  ICPrevOutput=DiscIntNeverNeededParam  ICPrevScaledInput=DiscIntNeverNeededParam
  Discrete-Time Integrator1 : DiscreteIntegrator  InitialCondition=init_state(8)  SampleTime=Ts_cal  ICPrevOutput=DiscIntNeverNeededParam  ICPrevScaledInput=DiscIntNeverNeededParam
  Gain : Gain  Gain=2*pi
  Gain1 : Gain  Gain=2*pi
  Product : Product  Inputs=3
  Product1 : Product  Inputs=3
  Product2 : Product
  Product3 : Product
  Scope : Scope
  Scope1 : Scope
  Square{,1..5} (6 alike) : Math  Operator=square  SaturateOnIntegerOverflow=on
  Subtract : Sum  Inputs=+-
  Subtract1 : Sum
  adaptive_f : MATLAB Function  TreatAsAtomicUnit=on
  u : Outport
  v : Outport  Port=2
  wires:
  f/1 -> [f]
  A/1 -> [A]
  k/1 -> [k]
  [A] -> Square/1
  [u] -> Square1/1
  [v] -> Square2/1
  Square2/1 -> Add/3
  Square1/1 -> Add/2
  Square/1 -> Add/1
  Add/1 -> Product/1
  [k] -> Product/2
  [u] -> Product/3
  Product/1 -> Subtract/1
  Square3/1 -> Add1/1
  Square4/1 -> Add1/2
  Square5/1 -> Add1/3
  [v] -> Product1/3
  Product1/1 -> Subtract1/1
  [v] -> Square5/1
  [A] -> Square3/1
  [u] -> Square4/1
  Add1/1 -> Product1/1
  [k] -> Product1/2
  [v] -> Product2/1
  [f_a] -> Product2/2
  Product2/1 -> Gain/1
  Gain/1 -> Subtract/2
  [u] -> Product3/1
  Product3/1 -> Gain1/1
  [f_a] -> Product3/2
  Gain1/1 -> Subtract1/2
  Subtract/1 -> Add2/2
  C/1 -> Demux/1
  Demux/1 -> [c_u]
  Demux/2 -> [c_v]
  [c_u] -> Add2/1
  Add2/1 -> Discrete-Time Integrator/1
  Subtract1/1 -> Add3/2
  [c_v] -> Add3/1
  alpha/1 -> [alpha]
  tau/1 -> [tau]
  [alpha] -> adaptive_f/1(alpha)
  [f] -> adaptive_f/2(f)
  [tau] -> adaptive_f/3(tau)
  [v] -> adaptive_f/4(v)
  adaptive_f/1(f_a) -> [f_a]
  Discrete-Time Integrator/1 -> u/1, Scope/1, [u]
  Add3/1 -> Discrete-Time Integrator1/1
  Discrete-Time Integrator1/1 -> v/1, Scope1/1, [v]

== system CPG_online/CPG/Subsystem ==
  alpha_r_vec : Inport
  alpha_b_vec : Inport  Port=2
  z_l_vec : Inport  Port=3
  Demux : Demux
  Demux1 : Demux
  Demux2 : Demux
  Mux{,6..8} (4 alike) : Mux  Inputs=3
  Mux5 : Mux
  Out1 : Outport
  wires:
  Mux6/1 -> Mux5/1
  Demux1/1 -> Mux6/2
  Demux/3 -> Mux8/1
  Demux2/1 -> Mux6/3
  alpha_b_vec/1 -> Demux1/1
  Demux/1 -> Mux6/1
  Demux2/4 -> Mux7/3
  Demux1/4 -> Mux7/2
  Demux/4 -> Mux7/1
  Mux5/1 -> Out1/1
  Demux2/3 -> Mux8/3
  Demux/2 -> Mux/1
  Mux8/1 -> Mux5/3
  Demux1/3 -> Mux8/2
  Demux1/2 -> Mux/2
  Mux7/1 -> Mux5/4
  Mux/1 -> Mux5/2
  Demux2/2 -> Mux/3
  z_l_vec/1 -> Demux2/1
  alpha_r_vec/1 -> Demux/1

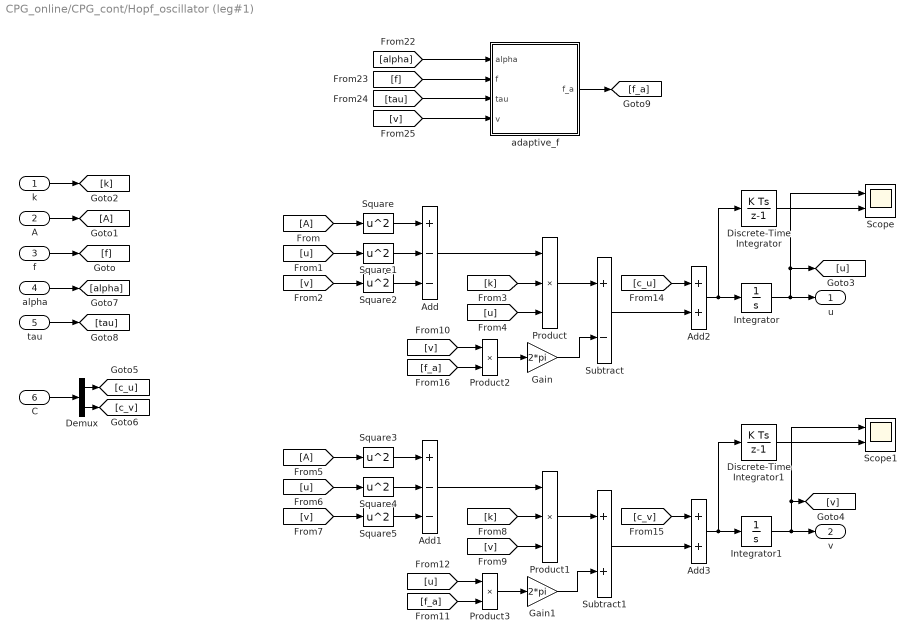
== system CPG_online/CPG_cont/Hopf_oscillator (leg#1) ==
  k : Inport
  A : Inport  Port=2
  f : Inport  Port=3
  alpha : Inport  Port=4
  tau : Inport  Port=5
  C : Inport  Port=6
  Add : Sum  Inputs=+--
  Add1 : Sum  Inputs=+--
  Add2 : Sum
  Add3 : Sum
  Demux : Demux  Outputs=2
  Discrete-Time Integrator : DiscreteIntegrator  InitialCondition=init_state(1)  SampleTime=Ts  ICPrevOutput=DiscIntNeverNeededParam  ICPrevScaledInput=DiscIntNeverNeededParam
  Discrete-Time Integrator1 : DiscreteIntegrator  InitialCondition=init_state(2)  SampleTime=Ts  ICPrevOutput=DiscIntNeverNeededParam  ICPrevScaledInput=DiscIntNeverNeededParam
  Gain : Gain  Gain=2*pi
  Gain1 : Gain  Gain=2*pi
  Integrator : Integrator  InitialCondition=init_state(1)
  Integrator1 : Integrator  InitialCondition=init_state(2)
  Product : Product  Inputs=3
  Product1 : Product  Inputs=3
  Product2 : Product
  Product3 : Product
  Scope : Scope  NumInputPorts=2
  Scope1 : Scope  NumInputPorts=2
  Square{,1..5} (6 alike) : Math  Operator=square  SaturateOnIntegerOverflow=on
  Subtract : Sum  Inputs=+-
  Subtract1 : Sum
  adaptive_f : MATLAB Function  TreatAsAtomicUnit=on
  u : Outport
  v : Outport  Port=2
  wires:
  Integrator/1 -> [u], Scope/1, u/1
  f/1 -> [f]
  A/1 -> [A]
  k/1 -> [k]
  [A] -> Square/1
  [u] -> Square1/1
  [v] -> Square2/1
  Square2/1 -> Add/3
  Square1/1 -> Add/2
  Square/1 -> Add/1
  Add/1 -> Product/1
  [k] -> Product/2
  [u] -> Product/3
  Product/1 -> Subtract/1
  Square3/1 -> Add1/1
  Square4/1 -> Add1/2
  Square5/1 -> Add1/3
  [v] -> Product1/3
  Product1/1 -> Subtract1/1
  [v] -> Square5/1
  [A] -> Square3/1
  [u] -> Square4/1
  Add1/1 -> Product1/1
  [k] -> Product1/2
  [v] -> Product2/1
  [f_a] -> Product2/2
  Product2/1 -> Gain/1
  Gain/1 -> Subtract/2
  [u] -> Product3/1
  Product3/1 -> Gain1/1
  [f_a] -> Product3/2
  Gain1/1 -> Subtract1/2
  Subtract/1 -> Add2/2
  C/1 -> Demux/1
  Demux/1 -> [c_u]
  Demux/2 -> [c_v]
  [c_u] -> Add2/1
  Add2/1 -> Discrete-Time Integrator/1, Integrator/1
  Subtract1/1 -> Add3/2
  [c_v] -> Add3/1
  Add3/1 -> Discrete-Time Integrator1/1, Integrator1/1
  alpha/1 -> [alpha]
  tau/1 -> [tau]
  [alpha] -> adaptive_f/1(alpha)
  [f] -> adaptive_f/2(f)
  [tau] -> adaptive_f/3(tau)
  [v] -> adaptive_f/4(v)
  adaptive_f/1(f_a) -> [f_a]
  Discrete-Time Integrator/1 -> Scope/2
  Discrete-Time Integrator1/1 -> Scope1/2
  Integrator1/1 -> Scope1/1, [v], v/1

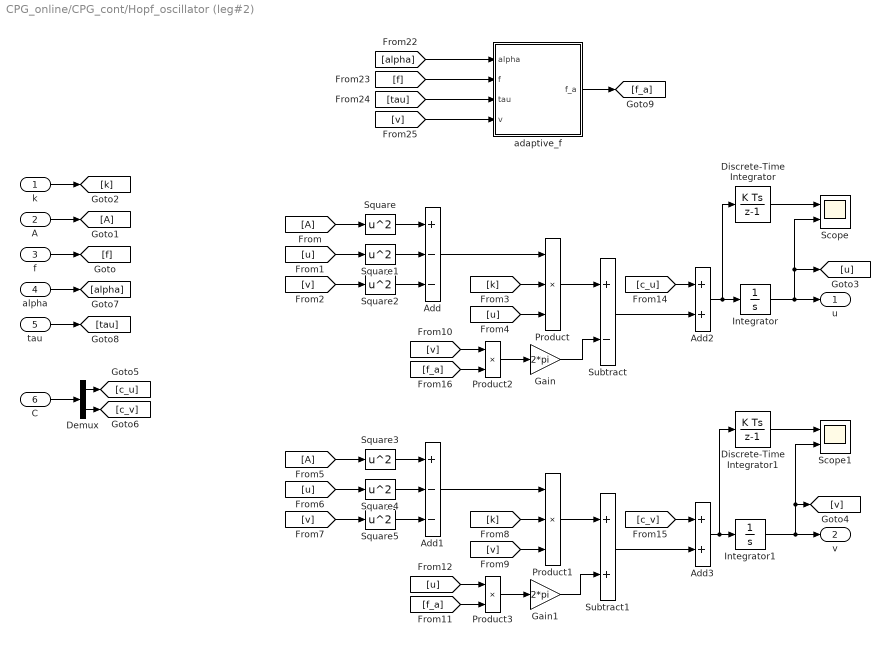
== system CPG_online/CPG_cont/Hopf_oscillator (leg#2) ==
  k : Inport
  A : Inport  Port=2
  f : Inport  Port=3
  alpha : Inport  Port=4
  tau : Inport  Port=5
  C : Inport  Port=6
  Add : Sum  Inputs=+--
  Add1 : Sum  Inputs=+--
  Add2 : Sum
  Add3 : Sum
  Demux : Demux  Outputs=2
  Discrete-Time Integrator : DiscreteIntegrator  InitialCondition=init_state(3)  SampleTime=Ts  ICPrevOutput=DiscIntNeverNeededParam  ICPrevScaledInput=DiscIntNeverNeededParam
  Discrete-Time Integrator1 : DiscreteIntegrator  InitialCondition=init_state(4)  SampleTime=Ts  ICPrevOutput=DiscIntNeverNeededParam  ICPrevScaledInput=DiscIntNeverNeededParam
  Gain : Gain  Gain=2*pi
  Gain1 : Gain  Gain=2*pi
  Integrator : Integrator  InitialCondition=init_state(3)
  Integrator1 : Integrator  InitialCondition=init_state(4)
  Product : Product  Inputs=3
  Product1 : Product  Inputs=3
  Product2 : Product
  Product3 : Product
  Scope : Scope  NumInputPorts=2
  Scope1 : Scope  NumInputPorts=2
  Square{,1..5} (6 alike) : Math  Operator=square  SaturateOnIntegerOverflow=on
  Subtract : Sum  Inputs=+-
  Subtract1 : Sum
  adaptive_f : MATLAB Function  TreatAsAtomicUnit=on
  u : Outport
  v : Outport  Port=2
  wires:
  f/1 -> [f]
  A/1 -> [A]
  k/1 -> [k]
  [A] -> Square/1
  [u] -> Square1/1
  [v] -> Square2/1
  Square2/1 -> Add/3
  Square1/1 -> Add/2
  Square/1 -> Add/1
  Add/1 -> Product/1
  [k] -> Product/2
  [u] -> Product/3
  Product/1 -> Subtract/1
  Square3/1 -> Add1/1
  Square4/1 -> Add1/2
  Square5/1 -> Add1/3
  [v] -> Product1/3
  Product1/1 -> Subtract1/1
  [v] -> Square5/1
  [A] -> Square3/1
  [u] -> Square4/1
  Add1/1 -> Product1/1
  [k] -> Product1/2
  [v] -> Product2/1
  [f_a] -> Product2/2
  Product2/1 -> Gain/1
  Gain/1 -> Subtract/2
  [u] -> Product3/1
  Product3/1 -> Gain1/1
  [f_a] -> Product3/2
  Gain1/1 -> Subtract1/2
  Subtract/1 -> Add2/2
  C/1 -> Demux/1
  Demux/1 -> [c_u]
  Demux/2 -> [c_v]
  [c_u] -> Add2/1
  Add2/1 -> Discrete-Time Integrator/1, Integrator/1
  Subtract1/1 -> Add3/2
  [c_v] -> Add3/1
  alpha/1 -> [alpha]
  tau/1 -> [tau]
  [alpha] -> adaptive_f/1(alpha)
  [f] -> adaptive_f/2(f)
  [tau] -> adaptive_f/3(tau)
  [v] -> adaptive_f/4(v)
  adaptive_f/1(f_a) -> [f_a]
  Discrete-Time Integrator/1 -> Scope/1
  Integrator/1 -> Scope/2, [u], u/1
  Discrete-Time Integrator1/1 -> Scope1/1
  Integrator1/1 -> Scope1/2, [v], v/1
  Add3/1 -> Discrete-Time Integrator1/1, Integrator1/1

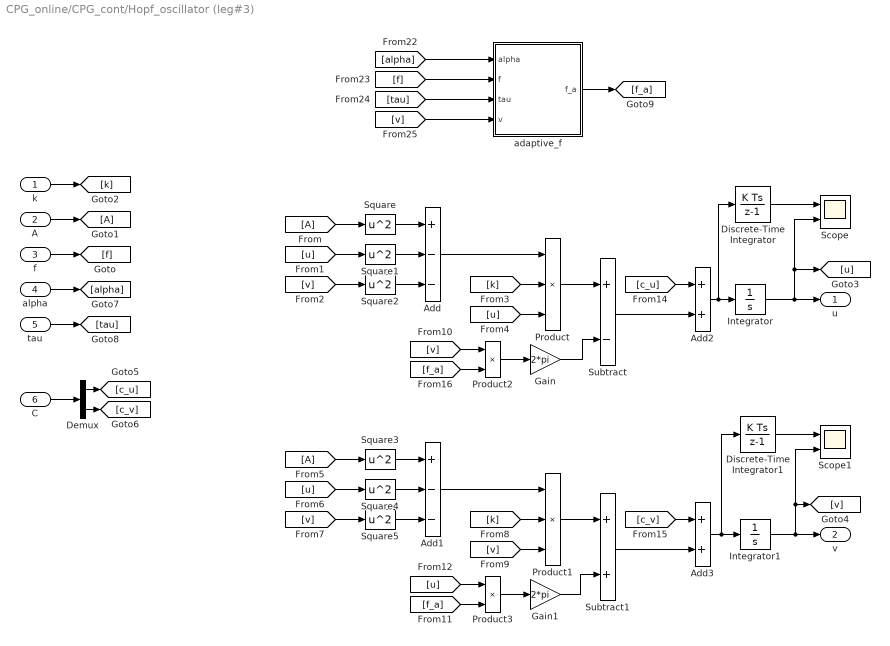
== system CPG_online/CPG_cont/Hopf_oscillator (leg#3) ==
  k : Inport
  A : Inport  Port=2
  f : Inport  Port=3
  alpha : Inport  Port=4
  tau : Inport  Port=5
  C : Inport  Port=6
  Add : Sum  Inputs=+--
  Add1 : Sum  Inputs=+--
  Add2 : Sum
  Add3 : Sum
  Demux : Demux  Outputs=2
  Discrete-Time Integrator : DiscreteIntegrator  InitialCondition=init_state(5)  SampleTime=Ts  ICPrevOutput=DiscIntNeverNeededParam  ICPrevScaledInput=DiscIntNeverNeededParam
  Discrete-Time Integrator1 : DiscreteIntegrator  InitialCondition=init_state(6)  SampleTime=Ts  ICPrevOutput=DiscIntNeverNeededParam  ICPrevScaledInput=DiscIntNeverNeededParam
  Gain : Gain  Gain=2*pi
  Gain1 : Gain  Gain=2*pi
  Integrator : Integrator  InitialCondition=init_state(5)
  Integrator1 : Integrator  InitialCondition=init_state(6)
  Product : Product  Inputs=3
  Product1 : Product  Inputs=3
  Product2 : Product
  Product3 : Product
  Scope : Scope  NumInputPorts=2
  Scope1 : Scope  NumInputPorts=2
  Square{,1..5} (6 alike) : Math  Operator=square  SaturateOnIntegerOverflow=on
  Subtract : Sum  Inputs=+-
  Subtract1 : Sum
  adaptive_f : MATLAB Function  TreatAsAtomicUnit=on
  u : Outport
  v : Outport  Port=2
  wires:
  Integrator/1 -> Scope/2, [u], u/1
  f/1 -> [f]
  A/1 -> [A]
  k/1 -> [k]
  [A] -> Square/1
  [u] -> Square1/1
  [v] -> Square2/1
  Square2/1 -> Add/3
  Square1/1 -> Add/2
  Square/1 -> Add/1
  Add/1 -> Product/1
  [k] -> Product/2
  [u] -> Product/3
  Product/1 -> Subtract/1
  Square3/1 -> Add1/1
  Square4/1 -> Add1/2
  Square5/1 -> Add1/3
  [v] -> Product1/3
  Product1/1 -> Subtract1/1
  [v] -> Square5/1
  [A] -> Square3/1
  [u] -> Square4/1
  Add1/1 -> Product1/1
  [k] -> Product1/2
  [v] -> Product2/1
  [f_a] -> Product2/2
  Product2/1 -> Gain/1
  Gain/1 -> Subtract/2
  [u] -> Product3/1
  Product3/1 -> Gain1/1
  [f_a] -> Product3/2
  Gain1/1 -> Subtract1/2
  Subtract/1 -> Add2/2
  C/1 -> Demux/1
  Demux/1 -> [c_u]
  Demux/2 -> [c_v]
  [c_u] -> Add2/1
  Add2/1 -> Discrete-Time Integrator/1, Integrator/1
  Subtract1/1 -> Add3/2
  [c_v] -> Add3/1
  Add3/1 -> Discrete-Time Integrator1/1, Integrator1/1
  alpha/1 -> [alpha]
  tau/1 -> [tau]
  [alpha] -> adaptive_f/1(alpha)
  [f] -> adaptive_f/2(f)
  [tau] -> adaptive_f/3(tau)
  [v] -> adaptive_f/4(v)
  adaptive_f/1(f_a) -> [f_a]
  Discrete-Time Integrator/1 -> Scope/1
  Discrete-Time Integrator1/1 -> Scope1/1
  Integrator1/1 -> Scope1/2, [v], v/1

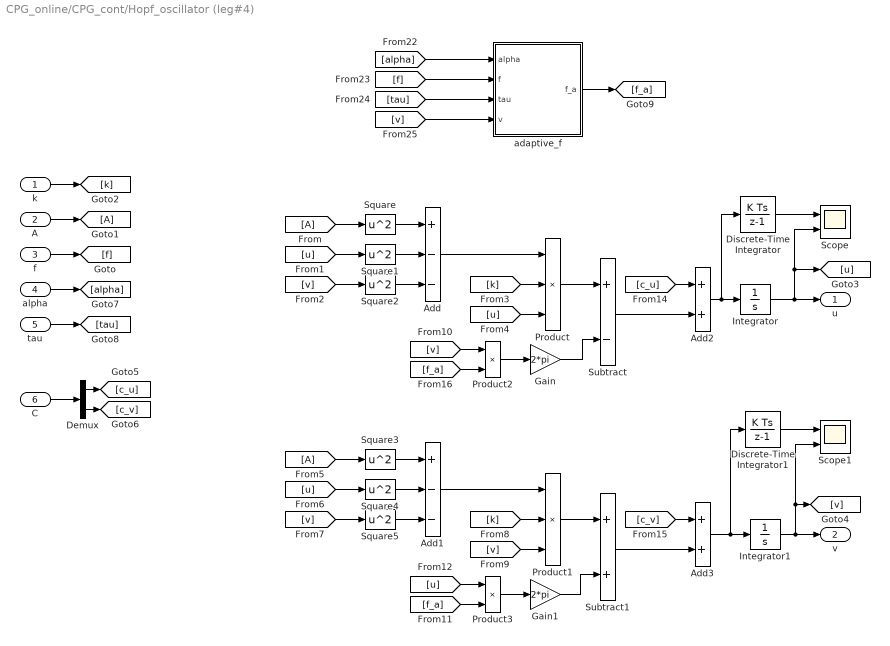
== system CPG_online/CPG_cont/Hopf_oscillator (leg#4) ==
  k : Inport
  A : Inport  Port=2
  f : Inport  Port=3
  alpha : Inport  Port=4
  tau : Inport  Port=5
  C : Inport  Port=6
  Add : Sum  Inputs=+--
  Add1 : Sum  Inputs=+--
  Add2 : Sum
  Add3 : Sum
  Demux : Demux  Outputs=2
  Discrete-Time Integrator : DiscreteIntegrator  InitialCondition=init_state(7)  SampleTime=Ts  ICPrevOutput=DiscIntNeverNeededParam  ICPrevScaledInput=DiscIntNeverNeededParam
  Discrete-Time Integrator1 : DiscreteIntegrator  InitialCondition=init_state(8)  SampleTime=Ts  ICPrevOutput=DiscIntNeverNeededParam  ICPrevScaledInput=DiscIntNeverNeededParam
  Gain : Gain  Gain=2*pi
  Gain1 : Gain  Gain=2*pi
  Integrator : Integrator  InitialCondition=init_state(7)
  Integrator1 : Integrator  InitialCondition=init_state(8)
  Product : Product  Inputs=3
  Product1 : Product  Inputs=3
  Product2 : Product
  Product3 : Product
  Scope : Scope  NumInputPorts=2
  Scope1 : Scope  NumInputPorts=2
  Square{,1..5} (6 alike) : Math  Operator=square  SaturateOnIntegerOverflow=on
  Subtract : Sum  Inputs=+-
  Subtract1 : Sum
  adaptive_f : MATLAB Function  TreatAsAtomicUnit=on
  u : Outport
  v : Outport  Port=2
  wires:
  f/1 -> [f]
  A/1 -> [A]
  k/1 -> [k]
  [A] -> Square/1
  [u] -> Square1/1
  [v] -> Square2/1
  Square2/1 -> Add/3
  Square1/1 -> Add/2
  Square/1 -> Add/1
  Add/1 -> Product/1
  [k] -> Product/2
  [u] -> Product/3
  Product/1 -> Subtract/1
  Square3/1 -> Add1/1
  Square4/1 -> Add1/2
  Square5/1 -> Add1/3
  [v] -> Product1/3
  Product1/1 -> Subtract1/1
  [v] -> Square5/1
  [A] -> Square3/1
  [u] -> Square4/1
  Add1/1 -> Product1/1
  [k] -> Product1/2
  [v] -> Product2/1
  [f_a] -> Product2/2
  Product2/1 -> Gain/1
  Gain/1 -> Subtract/2
  [u] -> Product3/1
  Product3/1 -> Gain1/1
  [f_a] -> Product3/2
  Gain1/1 -> Subtract1/2
  Subtract/1 -> Add2/2
  C/1 -> Demux/1
  Demux/1 -> [c_u]
  Demux/2 -> [c_v]
  [c_u] -> Add2/1
  Add2/1 -> Discrete-Time Integrator/1, Integrator/1
  Subtract1/1 -> Add3/2
  [c_v] -> Add3/1
  alpha/1 -> [alpha]
  tau/1 -> [tau]
  [alpha] -> adaptive_f/1(alpha)
  [f] -> adaptive_f/2(f)
  [tau] -> adaptive_f/3(tau)
  [v] -> adaptive_f/4(v)
  adaptive_f/1(f_a) -> [f_a]
  Discrete-Time Integrator/1 -> Scope/1
  Integrator/1 -> Scope/2, [u], u/1
  Add3/1 -> Discrete-Time Integrator1/1, Integrator1/1
  Integrator1/1 -> Scope1/2, [v], v/1
  Discrete-Time Integrator1/1 -> Scope1/1

== system CPG_online/CPG_cont/Subsystem ==
  alpha_r_vec : Inport
  alpha_b_vec : Inport  Port=2
  z_l_vec : Inport  Port=3
  Demux : Demux
  Demux1 : Demux
  Demux2 : Demux
  Mux{,6..8} (4 alike) : Mux  Inputs=3
  Mux5 : Mux
  Out1 : Outport
  wires:
  Mux6/1 -> Mux5/1
  Demux1/1 -> Mux6/2
  Demux/3 -> Mux8/1
  Demux2/1 -> Mux6/3
  alpha_b_vec/1 -> Demux1/1
  Demux/1 -> Mux6/1
  Demux2/4 -> Mux7/3
  Demux1/4 -> Mux7/2
  Demux/4 -> Mux7/1
  Mux5/1 -> Out1/1
  Demux2/3 -> Mux8/3
  Demux/2 -> Mux/1
  Mux8/1 -> Mux5/3
  Demux1/3 -> Mux8/2
  Demux1/2 -> Mux/2
  Mux7/1 -> Mux5/4
  Mux/1 -> Mux5/2
  Demux2/2 -> Mux/3
  z_l_vec/1 -> Demux2/1
  alpha_r_vec/1 -> Demux/1

== system CPG_online/Sensing/DataUnpack ==
  Byte Unpack{,1..14} (15 alike) : svdutilitieslib/Byte Unpack  dimensions={[1]}  datatypes={'single'}  byteAlign=1  blockPlatform=arduinoert
      settings: SourceProductBaseCode=ANDROID,ARDUINO,ML_ARDUINO,ECCORTEXA,ECCORTEXR,SC_BEAGLEBONE_BLUE,EC_FREEDOM_BOARD,EC_FRDM_K64F,INTEL_BLOCKSET,MICROBIT,NUCLEO,NVIDIA,PX4AUTOPILOTS,RASPPIIO,STMICRODIS,TIC2000,XILINX_BLOCKSET
  Cast To Double{,1..14} (15 alike) : DataTypeConversion  OutDataTypeStr=double
  Demux : Demux  Outputs=15
  TCP/IP Receive : instrumentlib/TCP//IP Receive  Priority=2  Host=192.168.0.111  Port=6666  DataSize=[60, 1 ]  DataType=uint8  ASCIIFormatting=%f  Terminator=LF  CustomTerminator=10  ByteOrder=big-endian  EnableBlockingMode=on  Timeout=1  SampleTime=Ts  SimulateUsing=Interpreted execution
  Front : Outport
  back : Outport  Port=2
  left : Outport  Port=3
  right : Outport  Port=4
  down : Outport  Port=5
  acc_x : Outport  Port=6
  acc_y : Outport  Port=7
  acc_z : Outport  Port=8
  FSR_FR : Outport  Port=9
  FSR_FL : Outport  Port=10
  FSR_RR : Outport  Port=11
  FSR_RL : Outport  Port=12
  rotx : Outport  Port=13
  roty : Outport  Port=14
  rotz : Outport  Port=15
  wires:
  Byte Unpack7/1 -> Cast To Double4/1
  Byte Unpack12/1 -> Cast To Double7/1
  Demux/5 -> Byte Unpack2/1
  Byte Unpack/1 -> Cast To Double9/1
  Byte Unpack6/1 -> Cast To Double3/1
  Demux/1 -> Byte Unpack12/1
  Demux/8 -> Byte Unpack5/1
  Demux/7 -> Byte Unpack4/1
  Demux/3 -> Byte Unpack/1
  Demux/4 -> Byte Unpack1/1
  Byte Unpack4/1 -> Cast To Double1/1
  Byte Unpack8/1 -> Cast To Double5/1
  Demux/6 -> Byte Unpack3/1
  Byte Unpack2/1 -> Cast To Double11/1
  Demux/2 -> Byte Unpack11/1
  Byte Unpack5/1 -> Cast To Double2/1
  Byte Unpack9/1 -> Cast To Double6/1
  Byte Unpack1/1 -> Cast To Double10/1
  Byte Unpack3/1 -> Cast To Double/1
  Byte Unpack11/1 -> Cast To Double8/1
  Cast To Double3/1 -> FSR_FR/1  "0~1"
  Cast To Double4/1 -> FSR_FL/1
  Cast To Double5/1 -> FSR_RR/1
  Cast To Double6/1 -> FSR_RL/1
  Cast To Double/1 -> rotx/1
  Cast To Double2/1 -> rotz/1
  Cast To Double1/1 -> roty/1
  Cast To Double7/1 -> Front/1  "Front"
  Cast To Double8/1 -> back/1  "back"
  Cast To Double9/1 -> left/1  "left"
  Cast To Double10/1 -> right/1  "right"
  Cast To Double11/1 -> down/1  "down"
  Demux/15 -> Byte Unpack9/1
  Demux/14 -> Byte Unpack8/1
  Demux/13 -> Byte Unpack7/1
  Demux/12 -> Byte Unpack6/1
  Cast To Double14/1 -> acc_z/1
  Byte Unpack10/1 -> Cast To Double12/1
  Cast To Double12/1 -> acc_x/1
  Cast To Double13/1 -> acc_y/1
  Byte Unpack13/1 -> Cast To Double13/1
  Byte Unpack14/1 -> Cast To Double14/1
  Demux/9 -> Byte Unpack10/1
  Demux/10 -> Byte Unpack13/1
  Demux/11 -> Byte Unpack14/1
  TCP/IP Receive/1 -> Demux/1

== system CPG_online/Sensing/rot_cal ==
  rotx_offset : Inport
  roty_offset : Inport  Port=2
  rotz_offset : Inport  Port=3
  euler : Inport  Port=4
  Add7 : Sum  Inputs=+-
  Add8 : Sum  Inputs=+-
  Add9 : Sum  Inputs=+-
  Demux1 : Demux  Outputs=3
  Subsystem : Subsystem
  Subsystem1 : Subsystem
  Subsystem2 : Subsystem
  rotz : Outport
  rotx : Outport  Port=2
  roty : Outport  Port=3
  wires:
  euler/1 -> Demux1/1  "rot"
  Add7/1 -> rotz/1  "rotz"
  rotz_offset/1 -> Add7/2
  Demux1/1 -> Subsystem2/1(rotx_raw)  "rotx"
  Demux1/2 -> Subsystem1/1(roty_raw)  "roty"
  Demux1/3 -> Subsystem/1(rotz_raw)  "rotz"
  roty_offset/1 -> Add8/2
  rotx_offset/1 -> Add9/2
  Add9/1 -> rotx/1  "rotx"
  Add8/1 -> roty/1  "roty"
  Subsystem/1(rotz) -> Add7/1
  Subsystem1/1(roty) -> Add8/1
  Subsystem2/1(rotx) -> Add9/1

== system CPG_online/Sensing/vx_cal ==
  front : Inport
  back : Inport  Port=2
  acc_x : Inport  Port=3
  Add : Sum  Inputs=+-
  Add1 : Sum  Inputs=+-
  Data Type Conversion1 : DataTypeConversion  OutDataTypeStr=double
  Data Type Conversion10 : DataTypeConversion  OutDataTypeStr=double
  Data Type Conversion9 : DataTypeConversion  OutDataTypeStr=double
  Delay : Delay  SampleTime=Ts
  Delay1 : Delay  DelayLength=1  SampleTime=Ts
  Delay2 : Delay  DelayLength=1  SampleTime=Ts
  Delay3 : Delay  DelayLength=1  InitialCondition=1500  SampleTime=Ts
  Gain : Gain  Gain=1/1000
  Gain12 : Gain  Gain=-1
  Kalman Filter : ctrlSharedLib/Kalman Filter  TimeDomain=Discrete-Time  UseCurrentEstimator=on  ModelSource=Individual A, B, C, D matrices  ModelSourceVariable=ss(0.95,1,1,0,1)  A=A  B=B  C=C  D=0  NumberOfStates=1  NumberOfInputs=1  NumberOfOutputs=1  InitialEstimateSource=Dialog  X0=[0;0]  P0=10  UseK=off  UseGH=off  NumberOfProcessNoiseInputs=1  G=1  TimeInvariantG=on  H=0  TimeInvariantH=on  Q=Q  TimeInvariantQ=on  R=R  TimeInvariantR=on  N=0  TimeInvariantN=on  AddInputPort=on  AddEnablePort=off  OutputEstimatedY=off  OutputP=off  Ts=Ts
  MATLAB Function : MATLAB Function  TreatAsAtomicUnit=on
  MATLAB Function1 : MATLAB Function  TreatAsAtomicUnit=on
  MATLAB Function2 : MATLAB Function  TreatAsAtomicUnit=on
  Terminator : Terminator
  vx : Outport
  wires:
  MATLAB Function/1(vx) -> Gain/1  "vx"
  Data Type Conversion9/1 -> Add1/1, Delay3/1  "v_front"
  Add1/1 -> Gain12/1
  front/1 -> Data Type Conversion9/1
  back/1 -> Data Type Conversion10/1
  Kalman Filter/1 -> MATLAB Function2/1(u)  "vx"
  acc_x/1 -> Data Type Conversion1/1
  Delay/1 -> MATLAB Function1/2(pred_acc), Delay1/1
  Delay1/1 -> MATLAB Function1/3(predd_acc)
  Data Type Conversion10/1 -> Delay2/1, Add/1  "v_back"
  Delay2/1 -> Add/2
  Add/1 -> MATLAB Function/2(v_back)
  Delay3/1 -> Add1/2
  MATLAB Function1/1(acceleration) -> Kalman Filter/1  "acc"
  MATLAB Function2/1(y) -> Terminator/1
  Data Type Conversion1/1 -> MATLAB Function1/1("acceleration "), Delay/1
  Gain12/1 -> MATLAB Function/1(v_front)
  MATLAB Function2/2(v) -> vx/1
  Gain/1 -> Kalman Filter/2  "vx"
